simulink model "a"  (R2020a)
settings: Solver=FixedStepAuto  StartTime=0.0  StopTime=10.68  FixedStep=0.01  RelTol=1e-3
undefined symbols (not defined in the file): a_PSM
settings Model: Creator=yizha  LastModifiedBy=Brock
settings DataIOCC: ReturnWorkspaceOutputs=off
settings DebuggingCC: ArithmeticOperatorsInVariantConditions=warning
settings SFSimCC: CustomCodeUndefinedFunction=UseInterfaceOnly

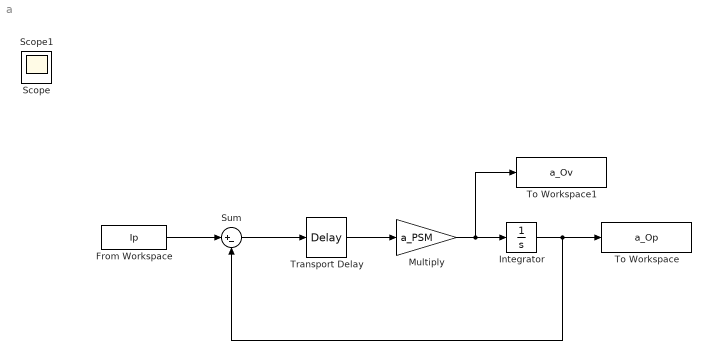
== system a ==
  From Workspace : FromWorkspace  VariableName=Ip
  Integrator : Integrator
  Multiply : Gain  Gain=a_PSM
  Sum : Sum  Inputs=|+-
  To Workspace : ToWorkspace  VariableName=a_Op  SaveFormat=Timeseries  SampleTime=-1
  To Workspace1 : ToWorkspace  VariableName=a_Ov  SaveFormat=Timeseries  SampleTime=-1
  Transport Delay : TransportDelay  DelayTime=0.1
  Scope : Scope
  Scope1 : Scope
  wires:
  From Workspace/1 -> Sum/1
  Sum/1 -> Transport Delay/1
  Transport Delay/1 -> Multiply/1
  Integrator/1 -> Sum/2, To Workspace/1
  Multiply/1 -> To Workspace1/1, Integrator/1
